simulink model "target_generation_test2"  (R2016b)
settings: Solver=VariableStepAuto  StartTime=0.0  StopTime=1000  RelTol=1e-3
values from neighbouring files (symbols this model uses):
  fsw_params = init_fsw_params()    [target_generation_test_init.m]
  sc_mode = 31    [target_generation_test_init.m]
libraries: aerolibutil x2, dynamics_lib x2, GPS_time_lib x1, pd_control_lib x1, aerolibtransform2 x1, RW_assembly_simple_lib x1, simulink_extras x1, MSP_FSW_lib x1, target_generation_lib x1, command_processing x1
settings Model: Creator=Taylor  LastModifiedBy=taylorreynolds

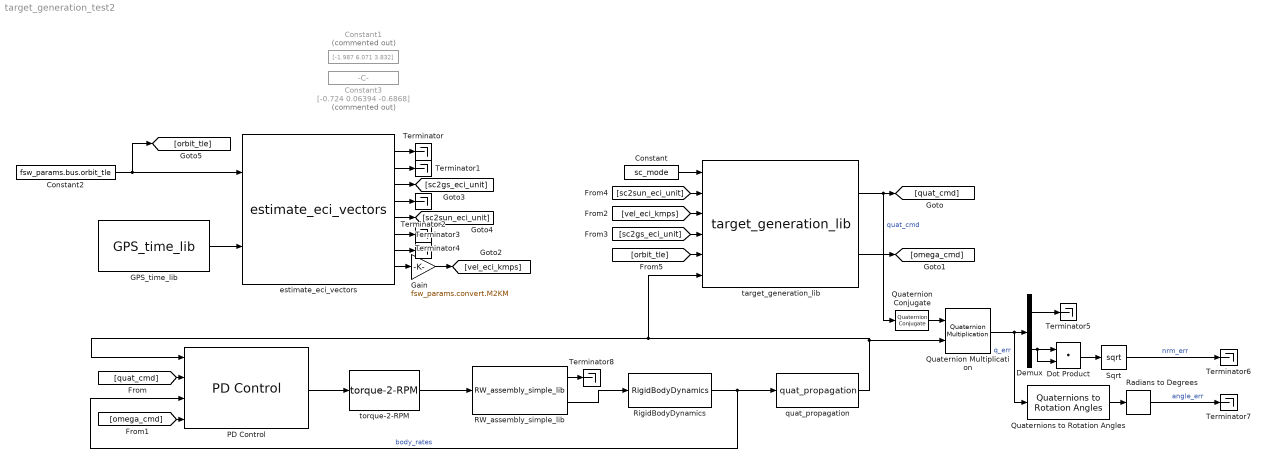
== system target_generation_test2 ==
  Constant : Constant  Value=sc_mode
  Constant1 : Constant  Commented=on  Value=[-1.987 6.071 3.832]
  Constant2 : Constant  Value=fsw_params.bus.orbit_tle
  Constant3 : Constant  Commented=on  Value=[-0.724 0.06394 -0.6868]
  Demux : Demux  Outputs=2
  Dot Product : DotProduct  InputSameDT=on  OutDataTypeStr=Inherit: Inherit via internal rule
  GPS_time_lib : GPS_time_lib/GPS_time_lib
  Gain : Gain  Gain=fsw_params.convert.M2KM
  PD Control : pd_control_lib/PD Control
  Quaternion Conjugate : aerolibutil/Quaternion Conjugate
  Quaternion Multiplication : aerolibutil/Quaternion Multiplication
  Quaternions to Rotation Angles : aerolibtransform2/Quaternions to Rotation Angles  rotationOrder=XYZ
  RW_assembly_simple_lib : RW_assembly_simple_lib/RW_assembly_simple_lib  natural_frequency=sim_params.actuators.reaction_wheel.natural_freq  damping_ratio=sim_params.actuators.reaction_wheel.damping  max_rate=sim_params.actuators.reaction_wheel.rate_limit
  Radians to Degrees : simulink_extras/Transformations/Radians to Degrees
  RigidBodyDynamics : dynamics_lib/Dynamics/RigidBodyDynamics
  Sqrt : Sqrt  SaturateOnIntegerOverflow=on
  Terminator{,1..8} (9 alike) : Terminator
  estimate_eci_vectors : MSP_FSW_lib/MSP_FSW/estimate_eci_vectors
  quat_propagation : dynamics_lib/Dynamics/quat_propagation
  target_generation_lib : target_generation_lib/target_generation_lib
  torque-2-RPM : command_processing/command_processing/torque-2-RPM
  wires:
  Constant/1 -> target_generation_lib/1
  Constant2/1 -> [orbit_tle], estimate_eci_vectors/1
  GPS_time_lib/1 -> estimate_eci_vectors/2
  RigidBodyDynamics/1 -> PD Control/3, quat_propagation/1  "body_rates"
  PD Control/1 -> torque-2-RPM/1
  quat_propagation/1 -> target_generation_lib/6, PD Control/1, Quaternion Multiplication/2
  estimate_eci_vectors/8 -> Gain/1
  target_generation_lib/1 -> Quaternion Conjugate/1, [quat_cmd]  "quat_cmd"
  target_generation_lib/2 -> [omega_cmd]
  [quat_cmd] -> PD Control/2
  [omega_cmd] -> PD Control/4
  Gain/1 -> [vel_eci_kmps]
  [vel_eci_kmps] -> target_generation_lib/3
  estimate_eci_vectors/1 -> Terminator/1
  estimate_eci_vectors/2 -> Terminator1/1
  estimate_eci_vectors/3 -> [sc2gs_eci_unit]
  [sc2gs_eci_unit] -> target_generation_lib/4
  estimate_eci_vectors/4 -> Terminator2/1
  estimate_eci_vectors/5 -> [sc2sun_eci_unit]
  [sc2sun_eci_unit] -> target_generation_lib/2
  estimate_eci_vectors/6 -> Terminator4/1
  estimate_eci_vectors/7 -> Terminator3/1
  [orbit_tle] -> target_generation_lib/5
  Quaternion Conjugate/1 -> Quaternion Multiplication/1
  Quaternion Multiplication/1 -> Quaternions to Rotation Angles/1, Demux/1  "q_err"
  Demux/1 -> Terminator5/1
  Demux/2 -> Dot Product/2, Dot Product/1
  Dot Product/1 -> Sqrt/1
  Sqrt/1 -> Terminator6/1  "nrm_err"
  Radians to Degrees/1 -> Terminator7/1  "angle_err"
  Quaternions to Rotation Angles/1 -> Radians to Degrees/1
  torque-2-RPM/1 -> RW_assembly_simple_lib/1
  RW_assembly_simple_lib/2 -> RigidBodyDynamics/1
  RW_assembly_simple_lib/1 -> Terminator8/1
